simulink model "SIMULINKSUSPENSION"  (R2024a)
settings: Solver=VariableStepAuto  StartTime=0.0  StopTime=10  RelTol=1e-3
InitFcn:
  | m1 = 290;
  | b1 = 1000;
  | m2 = 59;
  | k1 = 16182;
  | f = 0;
  | k2 = 19000;

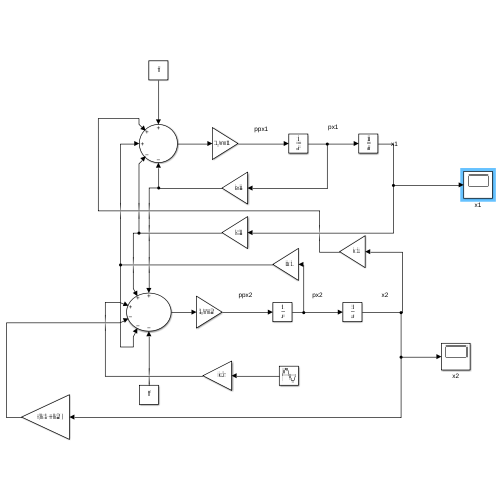
[thumbnail: Simulink's stored preview of the top-level diagram]
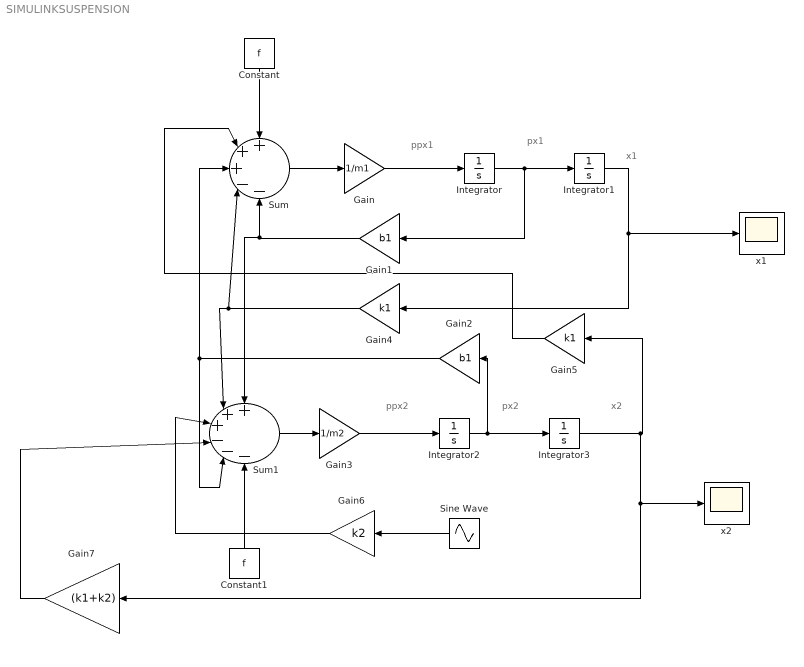
== system SIMULINKSUSPENSION ==
  note: x1
  note: px1
  note: ppx1
  note: ppx2
  note: x2
  note: px2
  Constant : Constant  Value=f
  Constant1 : Constant  Value=f
  Gain : Gain  Gain=1/m1
  Gain1 : Gain  Gain=b1
  Gain2 : Gain  Gain=b1
  Gain3 : Gain  Gain=1/m2
  Gain4 : Gain  Gain=k1
  Gain5 : Gain  Gain=k1
  Gain6 : Gain  Gain=k2
  Gain7 : Gain  Gain=(k1+k2)
  Integrator{,1..3} (4 alike) : Integrator
  Sine Wave : Sin  Amplitude=0.05  Frequency=0.5*pi  SampleTime=0
  Sum : Sum  Inputs=+++--
  Sum1 : Sum  Inputs=+++---
  x1 : Scope
  x2 : Scope
  wires:
  Integrator/1 -> Integrator1/1, Gain1/1
  Integrator1/1 -> Gain4/1, x1/1
  Gain/1 -> Integrator/1
  Sum/1 -> Gain/1
  Constant/1 -> Sum/1
  Gain1/1 -> Sum1/1, Sum/5
  Gain2/1 -> Sum1/5, Sum/3
  Gain3/1 -> Integrator2/1
  Integrator3/1 -> x2/1, Gain7/1, Gain5/1
  Integrator2/1 -> Integrator3/1, Gain2/1
  Gain5/1 -> Sum/2
  Constant1/1 -> Sum1/6
  Sum1/1 -> Gain3/1
  Gain6/1 -> Sum1/3
  Sine Wave/1 -> Gain6/1
  Gain4/1 -> Sum1/2, Sum/4
  Gain7/1 -> Sum1/4
